simulink model "Dome_Nov"  (R2022b)
settings: Solver=FixedStepAuto  StartTime=0  StopTime=5  FixedStep=Ts  RelTol=1e-3
undefined symbols (not defined in the file or in its folder): ApparatusDiscreDamping, ApparatusPara, ApparatusPowerFlow, ApparatusType, ListPowerFlowNew, OtherInputs, R, Ts, Wbase, x_e, Ybase, Zbase
libraries: spsGroundLib x12, SimplusGT x10, spsThreePhaseParallelRLCBranchLib x5, spsThreePhaseSeriesRLCBranchLib x3, spsControlledVoltageSourceLib x3, spsVoltageMeasurementLib x3, spsThreePhaseBreakerLib x2, sps_lib x1
settings Model: Creator=y_zhu  LastModifiedBy=yz34218

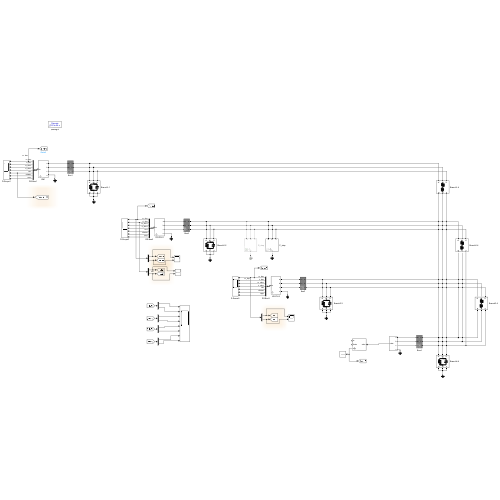
[thumbnail: Simulink's stored preview of the top-level diagram]
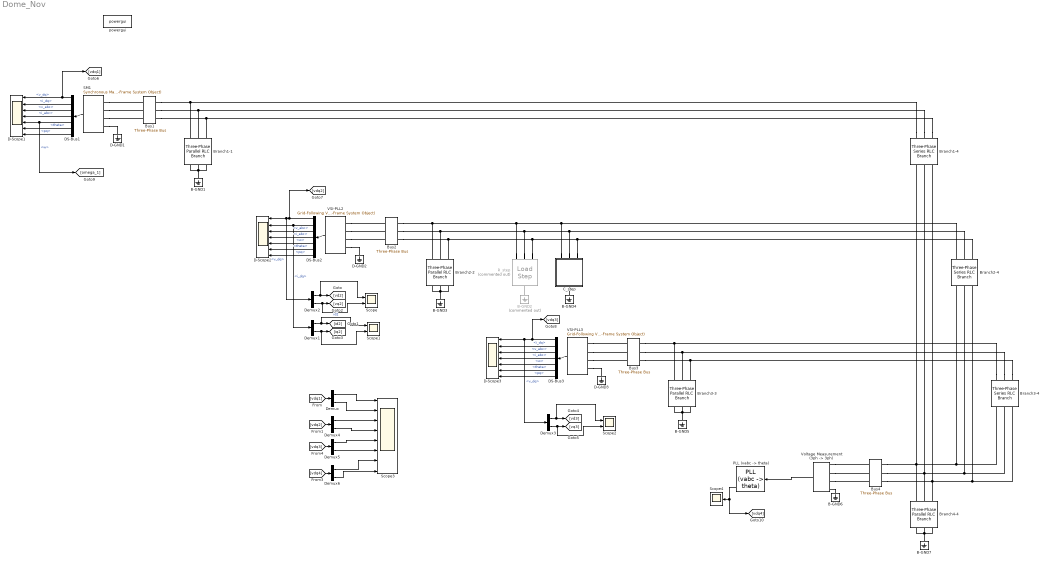
== system Dome_Nov ==
  B-GND{1,3..7} (6 alike) : spsGroundLib/Ground  LConnTagsString=a
  B-GND2 : spsGroundLib/Ground  Commented=on  LConnTagsString=a
  Branch1-1 : spsThreePhaseParallelRLCBranchLib/Three-Phase Parallel RLC Branch  LConnTagsString=A|B|C  RConnTagsString=A|B|C  BranchType=RC  Resistance=(1000000000)*Zbase  Inductance=(Inf)*Zbase/Wbase  Capacitance=(1e-09)*Ybase/Wbase  Measurements=None
  Branch1-4 : spsThreePhaseSeriesRLCBranchLib/Three-Phase Series RLC Branch  LConnTagsString=A|B|C  RConnTagsString=A|B|C  BranchType=RL  Resistance=(0.01)*Zbase  Inductance=(0.1)*Zbase/Wbase  Capacitance=1e-6  Measurements=None
  Branch2-2 : spsThreePhaseParallelRLCBranchLib/Three-Phase Parallel RLC Branch  LConnTagsString=A|B|C  RConnTagsString=A|B|C  BranchType=RC  Resistance=(13.8626)*Zbase  Inductance=(Inf)*Zbase/Wbase  Capacitance=(0.3)*Ybase/Wbase  Measurements=None
  Branch2-4 : spsThreePhaseSeriesRLCBranchLib/Three-Phase Series RLC Branch  LConnTagsString=A|B|C  RConnTagsString=A|B|C  BranchType=RL  Resistance=(0.03)*Zbase  Inductance=(0.3)*Zbase/Wbase  Capacitance=1e-6  Measurements=None
  Branch3-3 : spsThreePhaseParallelRLCBranchLib/Three-Phase Parallel RLC Branch  LConnTagsString=A|B|C  RConnTagsString=A|B|C  BranchType=RC  Resistance=(13.8626)*Zbase  Inductance=(Inf)*Zbase/Wbase  Capacitance=(0.3)*Ybase/Wbase  Measurements=None
  Branch3-4 : spsThreePhaseSeriesRLCBranchLib/Three-Phase Series RLC Branch  LConnTagsString=A|B|C  RConnTagsString=A|B|C  BranchType=RL  Resistance=(0.03)*Zbase  Inductance=(0.3)*Zbase/Wbase  Capacitance=1e-6  Measurements=None
  Branch4-4 : spsThreePhaseParallelRLCBranchLib/Three-Phase Parallel RLC Branch  LConnTagsString=A|B|C  RConnTagsString=A|B|C  BranchType=RC  Resistance=(11.3805)*Zbase  Inductance=(Inf)*Zbase/Wbase  Capacitance=(1e-09)*Ybase/Wbase  Measurements=None
  Bus{1..4} (4 alike) : SimplusGT/Three-Phase Bus  Vbase=1  Sbase=1
      settings: SourceProductName=Simplus Grid Tool
  C_step : Subsystem  AncestorBlock=SimplusGT/Load Step  mask{t0=3, C=(0.3)*Ybase/Wbase*0.01, Reverse=0}
      settings: LibrarySourceBlock=SimplusGT/Load Step
  D-GND1 : spsGroundLib/Ground  LConnTagsString=a
  D-GND2 : spsGroundLib/Ground  LConnTagsString=a
  D-GND3 : spsGroundLib/Ground  LConnTagsString=a
  D-Scope1 : Scope  NumInputPorts=7
  D-Scope2 : Scope  NumInputPorts=7
  D-Scope3 : Scope  NumInputPorts=7
  DS-Bus1 : BusSelector  OutputSignals=v_dq,i_dq,v_abc,i_abc,w,theta,pq
  DS-Bus2 : BusSelector  OutputSignals=v_dq,i_dq,v_abc,i_abc,w,theta,pq
  DS-Bus3 : BusSelector  OutputSignals=v_dq,i_dq,v_abc,i_abc,w,theta,pq
  Demux{,1..6} (7 alike) : Demux  Outputs=2
  "PLL (vabc -> theta)" : SimplusGT/PLL (vabc -> theta)  Ts=Ts  Wbase=Wbase  w_pll=2*pi*10  w_tau=2*pi*5  theta0=ListPowerFlowNew(4,5)
      settings: SourceProductName=Simplus Grid Tool
  R_step : SimplusGT/Load Step  Commented=on  t0=3  R=(13.8626)*Zbase*10  Reverse=0
      settings: SourceProductName=Simplus Grid Tool
  SM1 : SimplusGT/Synchronous Machine (dq-Frame System Object)  Ts=Ts  Sbase=Sbase  Vbase=Vbase  Wbase=Wbase  ApparatusType=ApparatusType{1}  ApparatusPara=ApparatusPara{1}  PowerFlow=ApparatusPowerFlow{1}  x0=x_e{1}  OtherInputs=OtherInputs{1}  DiscreMethod=Hybrid Trapezoidal  EnableInsideModification=off  DiscreDampingFlag=on  DiscreDampingValue=ApparatusDiscreDamping{1}  LinearizationTimes=1  DirectFeedthrough=off
      settings: SourceProductName=Simplus Grid Tool
  Scope : Scope  NumInputPorts=2
  Scope1 : Scope  NumInputPorts=2
  Scope2 : Scope  NumInputPorts=2
  Scope3 : Scope  NumInputPorts=8
  Scope4 : Scope
  VSI-PLL2 : SimplusGT/Grid-Following Voltage-Source Inverter (dq-Frame System Object)  Ts=Ts  Sbase=Sbase  Vbase=Vbase  Wbase=Wbase  ApparatusType=ApparatusType{2}  ApparatusPara=ApparatusPara{2}  PowerFlow=ApparatusPowerFlow{2}  x0=x_e{2}  OtherInputs=OtherInputs{2}  DiscreMethod=Hybrid Trapezoidal  EnableInsideModification=off  DiscreDampingFlag=on  DiscreDampingValue=ApparatusDiscreDamping{2}  LinearizationTimes=1  DirectFeedthrough=off
      settings: SourceProductName=Simplus Grid Tool
  VSI-PLL3 : SimplusGT/Grid-Following Voltage-Source Inverter (dq-Frame System Object)  Ts=Ts  Sbase=Sbase  Vbase=Vbase  Wbase=Wbase  ApparatusType=ApparatusType{3}  ApparatusPara=ApparatusPara{3}  PowerFlow=ApparatusPowerFlow{3}  x0=x_e{3}  OtherInputs=OtherInputs{3}  DiscreMethod=Hybrid Trapezoidal  EnableInsideModification=off  DiscreDampingFlag=on  DiscreDampingValue=ApparatusDiscreDamping{3}  LinearizationTimes=1  DirectFeedthrough=off
      settings: SourceProductName=Simplus Grid Tool
  "Voltage Measurement (3ph -> 3ph)" : SimplusGT/Voltage Measurement (3ph -> 3ph)  SystemSampleTime=-1  VariantActivationTime=update diagram  Latency=0  AutoFrameSizeCalculation=off
      settings: SourceProductName=Simplus Grid Tool
  powergui : sps_lib/powergui  Priority=1  SimulationMode=Discrete  SampleTime=Ts  frequency=60  Iterations=50  frequencyindice=0  Pbase=100e6  ErrMax=1e-4  UnitsV=kV  UnitsW=MW  buscounter=0  FunctionMessages=off  echomessages=off  EnableUseOfTLC=off  CurrentSourceSwitches=off  DisableSnubberDevices=off  DisableRonSwitches=off  DisableVfSwitches=off  DisplayEquations=off  AutomaticDiscreteSolvers=off  SolverType=Tustin/Backward Euler (TBE)  Interpol=off  ExternalGateDelay=off  methode=off  Ts=100  x0status=blocks  SPID=on  SwTol=0  HookPort=off  NonlinearTolerance=1e-4  nMaxIteration=100  ContinueOnMaxIteration=off  RestoreLinks=warning  ResistiveCurrentMeasurement=off  Frange=[0:2:500]  Ylog=off  Xlog=on  ShowGrid=off  save=off  variable=ZData  structure=0  ZoomFFT=off  StartTime=0.0  cycles=1  DisplayStyle=1  fundamental=60  FreqAxis=off  MaxFrequency=1000  frequencyindicesteady=1  RmsSteady=1  display=off
  wires:
  SM1/1 -> DS-Bus1/1
  DS-Bus1/2 -> D-Scope1/2  "<i_dq>"
  DS-Bus1/3 -> D-Scope1/3  "<v_abc>"
  DS-Bus1/4 -> D-Scope1/4  "<i_abc>"
  DS-Bus1/5 -> [omega_1], D-Scope1/5  "<w>"
  DS-Bus1/6 -> D-Scope1/6  "<theta>"
  DS-Bus1/7 -> D-Scope1/7  "<pq>"
  VSI-PLL2/1 -> DS-Bus2/1
  DS-Bus2/1 -> [vdq2], Demux2/1, D-Scope2/1  "<v_dq>"
  DS-Bus2/2 -> Demux1/1, D-Scope2/2  "<i_dq>"
  DS-Bus2/3 -> D-Scope2/3  "<v_abc>"
  DS-Bus2/4 -> D-Scope2/4  "<i_abc>"
  DS-Bus2/5 -> D-Scope2/5  "<w>"
  DS-Bus2/6 -> D-Scope2/6  "<theta>"
  DS-Bus2/7 -> D-Scope2/7  "<pq>"
  VSI-PLL3/1 -> DS-Bus3/1
  DS-Bus3/2 -> D-Scope3/2  "<i_dq>"
  DS-Bus3/3 -> D-Scope3/3  "<v_abc>"
  DS-Bus3/4 -> D-Scope3/4  "<i_abc>"
  DS-Bus3/5 -> D-Scope3/5  "<w>"
  DS-Bus3/6 -> D-Scope3/6  "<theta>"
  DS-Bus3/7 -> D-Scope3/7  "<pq>"
  Demux2/1 -> Scope/1, [vd2]
  Demux1/1 -> Scope1/1, [id2]  "id2"
  Demux2/2 -> Scope/2, [vq2]
  Demux1/2 -> Scope1/2, [iq2]
  Demux3/1 -> Scope2/1, [vd3]
  DS-Bus3/1 -> [vdq3], Demux3/1, D-Scope3/1  "<v_dq>"
  Demux3/2 -> Scope2/2, [vq3]
  DS-Bus1/1 -> [vdq1], D-Scope1/1  "<v_dq>"
  "Voltage Measurement (3ph -> 3ph)"/1 -> "PLL (vabc -> theta)"/1
  "PLL (vabc -> theta)"/3 -> [vdq4], Scope4/1
  [vdq1] -> Demux/1
  [vdq2] -> Demux4/1
  [vdq3] -> Demux5/1
  [vdq4] -> Demux6/1
  Demux/1 -> Scope3/1
  Demux/2 -> Scope3/2
  Demux4/1 -> Scope3/3
  Demux4/2 -> Scope3/4
  Demux5/1 -> Scope3/5
  Demux5/2 -> Scope3/6
  Demux6/1 -> Scope3/7
  Demux6/2 -> Scope3/8
  connections:
  SM1/LConn4 -- D-GND1/LConn1
  VSI-PLL2/LConn4 -- D-GND2/LConn1
  VSI-PLL3/LConn4 -- D-GND3/LConn1
  Branch1-1/RConn1 -- Branch1-1/RConn2 -- Branch1-1/RConn3 -- B-GND1/LConn1
  Branch2-2/RConn1 -- Branch2-2/RConn2 -- Branch2-2/RConn3 -- B-GND3/LConn1
  Branch3-3/RConn1 -- Branch3-3/RConn2 -- Branch3-3/RConn3 -- B-GND5/LConn1
  Branch4-4/RConn1 -- Branch4-4/RConn2 -- Branch4-4/RConn3 -- B-GND7/LConn1
  Branch1-4/RConn1 -- Bus4/RConn1 -- Branch4-4/LConn1 -- Branch3-4/RConn1 -- Branch2-4/RConn1
  Branch1-4/RConn2 -- Bus4/RConn2 -- Branch4-4/LConn2 -- Branch3-4/RConn2 -- Branch2-4/RConn2
  Branch1-4/RConn3 -- Bus4/RConn3 -- Branch4-4/LConn3 -- Branch3-4/RConn3 -- Branch2-4/RConn3
  Branch1-4/LConn1 -- Bus1/RConn1 -- Branch1-1/LConn1
  Branch1-4/LConn2 -- Bus1/RConn2 -- Branch1-1/LConn2
  Branch1-4/LConn3 -- Bus1/RConn3 -- Branch1-1/LConn3
  Bus2/RConn1 -- Branch2-2/LConn1 -- R_step/LConn1 -- Branch2-4/LConn1 -- C_step/LConn1
  Bus2/RConn2 -- Branch2-2/LConn2 -- R_step/LConn2 -- Branch2-4/LConn2 -- C_step/LConn2
  Bus2/RConn3 -- Branch2-2/LConn3 -- R_step/LConn3 -- Branch2-4/LConn3 -- C_step/LConn3
  Branch3-4/LConn1 -- Bus3/RConn1 -- Branch3-3/LConn1
  Branch3-4/LConn2 -- Bus3/RConn2 -- Branch3-3/LConn2
  Branch3-4/LConn3 -- Bus3/RConn3 -- Branch3-3/LConn3
  SM1/LConn1 -- Bus1/LConn1
  SM1/LConn2 -- Bus1/LConn2
  SM1/LConn3 -- Bus1/LConn3
  VSI-PLL2/LConn1 -- Bus2/LConn1
  VSI-PLL2/LConn2 -- Bus2/LConn2
  VSI-PLL2/LConn3 -- Bus2/LConn3
  VSI-PLL3/LConn1 -- Bus3/LConn1
  VSI-PLL3/LConn2 -- Bus3/LConn2
  VSI-PLL3/LConn3 -- Bus3/LConn3
  B-GND2/LConn1 -- R_step/RConn1
  B-GND4/LConn1 -- C_step/RConn1
  "Voltage Measurement (3ph -> 3ph)"/LConn1 -- Bus4/LConn1
  "Voltage Measurement (3ph -> 3ph)"/LConn2 -- Bus4/LConn2
  "Voltage Measurement (3ph -> 3ph)"/LConn3 -- Bus4/LConn3
  "Voltage Measurement (3ph -> 3ph)"/LConn4 -- B-GND6/LConn1

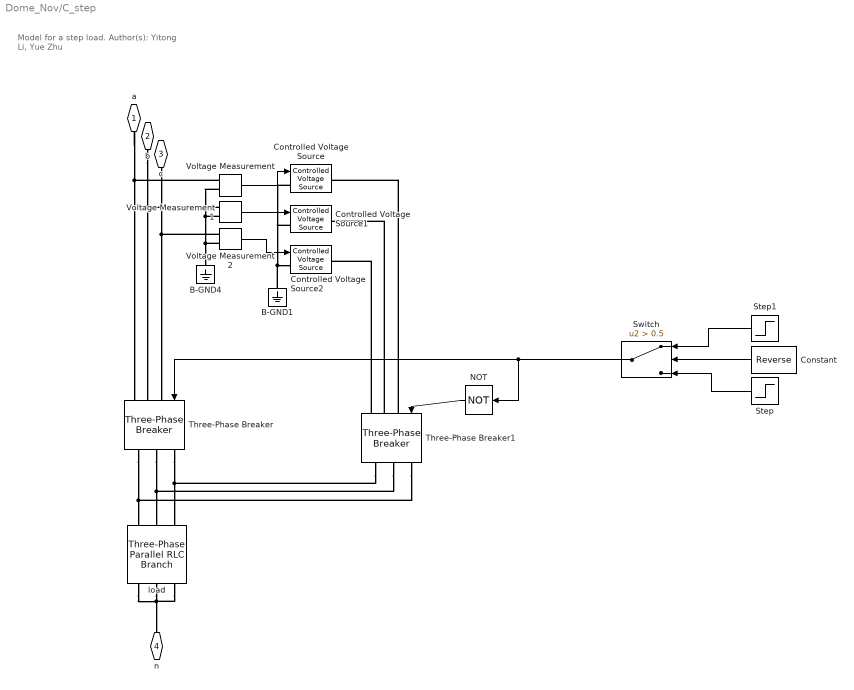
== system Dome_Nov/C_step ==
  note: Model for a step load.
      |
      | Author(s): Yitong Li, Yue Zhu
  B-GND1 : spsGroundLib/Ground  LConnTagsString=a
  B-GND4 : spsGroundLib/Ground  LConnTagsString=a
  Constant : Constant  Value=Reverse
  Controlled Voltage Source : spsControlledVoltageSourceLib/Controlled Voltage Source  Initialize=on  Source_Type=AC  Amplitude=0  Phase=0  Frequency=0  Measurements=None
  Controlled Voltage Source1 : spsControlledVoltageSourceLib/Controlled Voltage Source  Initialize=on  Source_Type=AC  Amplitude=0  Phase=0  Frequency=0  Measurements=None
  Controlled Voltage Source2 : spsControlledVoltageSourceLib/Controlled Voltage Source  Initialize=on  Source_Type=AC  Amplitude=0  Phase=0  Frequency=0  Measurements=None
  NOT : Logic  Operator=NOT  IconShape=distinctive  AllPortsSameDT=off  OutDataTypeStr=boolean
  Step : Step  Time=t0  SampleTime=0
  Step1 : Step  Time=t0  Before=1  After=0  SampleTime=0
  Switch : Switch  Criteria=u2 > Threshold  Threshold=0.5  SaturateOnIntegerOverflow=off  InputSameDT=off
  Three-Phase Breaker : spsThreePhaseBreakerLib/Three-Phase Breaker  InitialState=open  SwitchA=on  SwitchB=on  SwitchC=on  SwitchTimes="[1/60  5/60]"  External=on  BreakerResistance=0.01  SnubberResistance=1e6  SnubberCapacitance=inf  Measurements=None
  Three-Phase Breaker1 : spsThreePhaseBreakerLib/Three-Phase Breaker  InitialState=open  SwitchA=on  SwitchB=on  SwitchC=on  SwitchTimes="[1/60  5/60]"  External=on  BreakerResistance=0.01  SnubberResistance=1e6  SnubberCapacitance=inf  Measurements=None
  Voltage Measurement : spsVoltageMeasurementLib/Voltage Measurement  PhasorSimulation=off  OutputType=Complex  PSBequivalent=0
  Voltage Measurement1 : spsVoltageMeasurementLib/Voltage Measurement  PhasorSimulation=off  OutputType=Complex  PSBequivalent=0
  Voltage Measurement2 : spsVoltageMeasurementLib/Voltage Measurement  PhasorSimulation=off  OutputType=Complex  PSBequivalent=0
  load : spsThreePhaseParallelRLCBranchLib/Three-Phase Parallel RLC Branch  LConnTagsString=A|B|C  RConnTagsString=A|B|C  BranchType=C  Resistance=R  Inductance=1  Capacitance=C  Measurements=None
  a : PMIOPort  Side=Left
  b : PMIOPort  Port=2  Side=Left
  c : PMIOPort  Port=3  Side=Left
  n : PMIOPort  Port=4  Side=Right
  wires:
  Step/1 -> Switch/3
  Step1/1 -> Switch/1
  Constant/1 -> Switch/2
  Switch/1 -> NOT/1, Three-Phase Breaker/1
  Voltage Measurement/1 -> Controlled Voltage Source/1
  Voltage Measurement1/1 -> Controlled Voltage Source1/1
  Voltage Measurement2/1 -> Controlled Voltage Source2/1
  NOT/1 -> Three-Phase Breaker1/1
  connections:
  c/RConn1 -- Voltage Measurement2/LConn1 -- Three-Phase Breaker/LConn1
  Three-Phase Breaker/RConn1 -- Three-Phase Breaker1/RConn3 -- load/LConn3
  load/RConn1 -- load/RConn3 -- n/RConn1 -- load/RConn2
  Three-Phase Breaker/RConn2 -- Three-Phase Breaker1/RConn2 -- load/LConn2
  Three-Phase Breaker/RConn3 -- Three-Phase Breaker1/RConn1 -- load/LConn1
  b/RConn1 -- Three-Phase Breaker/LConn2 -- Voltage Measurement1/LConn1
  a/RConn1 -- Voltage Measurement/LConn1 -- Three-Phase Breaker/LConn3
  Voltage Measurement/LConn2 -- Voltage Measurement1/LConn2 -- Voltage Measurement2/LConn2 -- B-GND4/LConn1
  B-GND1/LConn1 -- Controlled Voltage Source1/LConn1 -- Controlled Voltage Source/LConn1 -- Controlled Voltage Source2/LConn1
  Three-Phase Breaker1/LConn1 -- Controlled Voltage Source/RConn1
  Three-Phase Breaker1/LConn2 -- Controlled Voltage Source1/RConn1
  Three-Phase Breaker1/LConn3 -- Controlled Voltage Source2/RConn1
